simulink model "ModelForSlidesFeb"  (R2023a)
settings: Solver=VariableStepAuto  StartTime=0  StopTime=1000  FixedStep=0.01  RelTol=1e-3
model workspace (MAT data in the model file):
  finalint = 0
  firstWarning = 1
  originalScenarioChecksum = '114339432DE22364D47BB28FC96DC10C'
undefined symbols (not defined in the file): Acceleration, ActorID, AngularVelocity, curvature, DefaultGear, Defined, DEND_B, DEND_S, DEND_T, direction, DiscIntNeverNeededParam, driving, Ego, gradbp, L, Lane, LF, LR, m, matlabshared, MAX_BRAKE, MAX_STEER, MAX_TORQUE, maxNumActors, MCAR, MIN_BRAKE, MIN_STEER, MIN_TORQUE, n, NUMD_B, NUMD_S, NUMD_T, Pitch, Pose, Position, psi_o, R, Roll, RRdamp, SceneInfo, session, sigbuilder_block, STEER_RATIO, stopSign_ID, Tdead, thetaRefs, TL_ID, TrackWidth, ts, Ts, User, Vdead, Velocity, WB, X_o, xRef2s, Y_o, Yaw, yRef2s
libraries: drivingscenarioandsensors x13, roadrunnerscenario x11, simulink x8, simulink_extras x5, drivingvehiclecontroller x2, trackingutilitieslib x2, robotalgslib x1, mpcadaslib x1, slpidlib x1, drivinglib x1, autolibshared x1, vehdynlibviscommon x1
(part 1 of 4)
settings Model: Creator=akshran  LastModifiedBy=almudhaf.3
settings DataIOCC: SignalLogging=off
settings OptimizationCC: ReuseModelBlockBuffer=off
settings DebuggingCC: UnconnectedInputMsg=warning  UnconnectedOutputMsg=warning  UnconnectedLineMsg=warning  UnderSpecifiedDimensionMsg=warning
settings ModelReferenceCC: EnableRefExpFcnMdlSchedulingChecks=on
settings RTWCC: DLArmComputeVersion=19.05

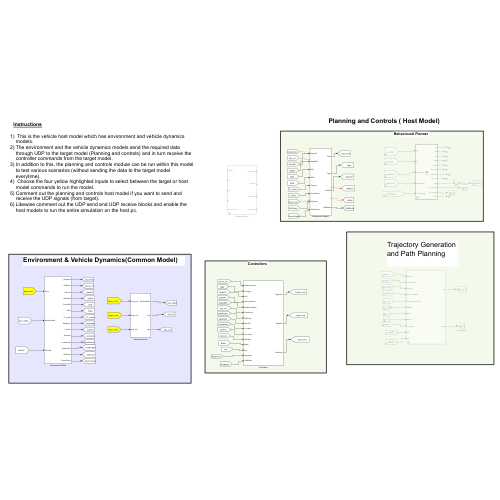
[thumbnail: Simulink's stored preview of the top-level diagram]
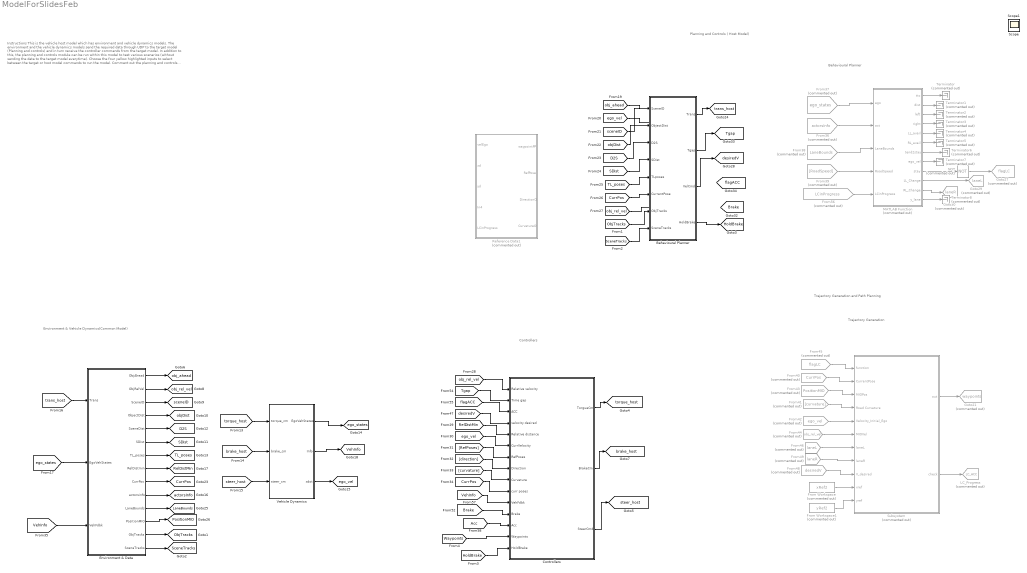
== system ModelForSlidesFeb ==
  note: Trajectory Generation and Path Planning
  note: Trajectory Generation
  note: Behavioural Planner
  note: Instructions
      |
      | This is the vehicle host model which has environment and vehicle dynamics models.
      | The environment and the vehicle dynamics models send the required data through UDP to the target model (Planning and controls) and in turn receive the controller commands from the target model.
      | In addition to this, the planning and controls module can be run within this model to test various scenarios (without sending the data to the target model everytime).
      | Choose the four yellow highlighted inputs to select between the target or host model commands to run the model.
      | Comment out the planning and controls host model if you want to send and receive the UDP signals (from target).
      | Likewise comment out the UDP send and UDP receive blocks and enable the host models to run the entire simulation on the host pc.
  note: Environment & Vehicle Dynamics(Common Model)
  note: Planning and Controls ( Host Model)
  note: Controllers
  Behavioural Planner : Subsystem
  Controllers : Subsystem
  Environment & Data : Subsystem
  From Workspace : FromWorkspace  Commented=on  VariableName=xRef2
  From Workspace1 : FromWorkspace  Commented=on  VariableName=yRef2
  From36 : From  Commented=on  GotoTag=actorsInfo  TagVisibility=global
  From37 : From  Commented=on  GotoTag=ego_states  TagVisibility=global
  From38 : From  Commented=on  GotoTag=LaneBounds  TagVisibility=global
  From39 : From  Commented=on  GotoTag=RoadSpeed  TagVisibility=global
  From40 : From  Commented=on  GotoTag=CurrPos  TagVisibility=global
  From41 : From  Commented=on  GotoTag=curvature
  From42 : From  Commented=on  GotoTag=ego_vel  TagVisibility=global
  From43 : From  Commented=on  GotoTag=PositionMIO  TagVisibility=global
  From44 : From  Commented=on  GotoTag=obj_rel_vel  TagVisibility=global
  From45 : From  Commented=on  GotoTag=flagLC  TagVisibility=global
  From46 : From  Commented=on  GotoTag=laneL  TagVisibility=global
  From48 : From  Commented=on  GotoTag=desiredV  TagVisibility=global
  From49 : From  Commented=on  GotoTag=laneR  TagVisibility=global
  From56 : From  Commented=on  GotoTag=LCinProgress  TagVisibility=global
  Goto21 : Goto  Commented=on  GotoTag=waypoints  TagVisibility=global
  Goto27 : Goto  Commented=on  GotoTag=flagLC  TagVisibility=global
  Goto29 : Goto  Commented=on  GotoTag=laneL  TagVisibility=global
  Goto30 : Goto  Commented=on  GotoTag=laneR  TagVisibility=global
  LC_Progress : Goto  Commented=on  GotoTag=LC_ACC  TagVisibility=global
  MATLAB Function : MATLAB Function  Commented=on  TreatAsAtomicUnit=on
  NOT : Logic  Commented=on  Operator=NOT  IconShape=distinctive  AllPortsSameDT=off  OutDataTypeStr=boolean
  Reference Data1 : Subsystem  Commented=on  VariantControl=Stanley
  Subsystem : Subsystem  Commented=on
  Terminator{,1..8} (9 alike) : Terminator  Commented=on
  Vehicle Dynamics : Subsystem
  Scope : Scope
  Scope1 : Scope
  tag scope: Brake=global, CurrPos=global, D2S=global, HoldBrake=global, LaneBounds=global, ObjTracks=global, PositionMIO=global, RelDistMin=global, SDist=global, SceneTracks=global, TL_poses=global, Tgap=global, VehInfo=global, actorsInfo=global, brake_host=global, desiredV=global, ego_states=global, ego_vel=global, flagACC=global, objDist=global, obj_ahead=global, obj_rel_vel=global, sceneID=global, steer_host=global, torque_host=global, trans_host=global
  wires:
  Controllers/1(TorgueCm) -> [torque_host]
  Environment & Data/1(ObjAhead) -> [obj_ahead]
  Environment & Data/2(ObjRelVel) -> [obj_rel_vel]
  Environment & Data/3(SceneID) -> [sceneID]
  Environment & Data/4(ObjectDist) -> [objDist]
  Environment & Data/6(SDist) -> [SDist]
  Environment & Data/5(SceneDist) -> [D2S]
  Environment & Data/7(TL_poses) -> [TL_poses]
  Vehicle Dynamics/1(EgoVehStates) -> [ego_states]
  Vehicle Dynamics/3(xdot) -> [ego_vel]
  Environment & Data/8(RelDistmin) -> [RelDistMin]
  Vehicle Dynamics/2(Info) -> [VehInfo]
  [torque_host] -> Vehicle Dynamics/1(torque_cm)
  [brake_host] -> Vehicle Dynamics/2(brake_cm)
  [steer_host] -> Vehicle Dynamics/3(steer_cm)
  [trans_host] -> Environment & Data/1(Trans)
  [ego_states] -> Environment & Data/2(EgoVehStates)
  [obj_rel_vel] -> Controllers/1(Relative velocity)
  [RelDistMin] -> Controllers/5(Relative distance)
  [ego_vel] -> Controllers/6(CurrVelocity)
  [RefPoses] -> Controllers/7(RefPoses)
  [direction] -> Controllers/8(Direction)
  [curvature] -> Controllers/9(Curvature)
  [CurrPos] -> Controllers/10(curr poses)
  [VehInfo] -> Environment & Data/3(VehFdbk)
  Environment & Data/9(CurrPos) -> [CurrPos]
  Environment & Data/10(actorsinfo) -> [actorsInfo]
  From37/1 -> MATLAB Function/1(ego)
  From36/1 -> MATLAB Function/2(act)
  Environment & Data/11(LaneBounds) -> [LaneBounds]
  From38/1 -> MATLAB Function/3(LaneBounds)
  From39/1 -> MATLAB Function/4(RoadSpeed)
  MATLAB Function/9(stay) -> NOT/1
  MATLAB Function/10(LL_Change) -> Goto29/1
  MATLAB Function/11(RL_Change) -> Goto30/1
  Environment & Data/12(PositionMIO) -> [PositionMIO]
  NOT/1 -> Goto27/1
  [desiredV] -> Controllers/4(velocity desired)
  [Tgap] -> Controllers/2(Time gap)
  [flagACC] -> Controllers/3(ACC)
  From56/1 -> MATLAB Function/5(LCinProgress)
  [VehInfo] -> Controllers/11(VehFdbk)
  Controllers/2(BrakeCm) -> [brake_host]
  Controllers/3(SteerCmd) -> [steer_host]
  From45/1 -> Subsystem/1(function)
  From40/1 -> Subsystem/2(CurrentPose)
  From43/1 -> Subsystem/3(MIOPos)
  From41/1 -> Subsystem/4(Road Curvature)
  From42/1 -> Subsystem/5(Velocity_Initial_Ego)
  From44/1 -> Subsystem/6(MIOVel)
  From48/1 -> Subsystem/9(V_desired)
  Subsystem/2(check) -> LC_Progress/1
  [obj_ahead] -> ?
  [ego_vel] -> ?
  [sceneID] -> Behavioural Planner/1(SceneID)
  [objDist] -> Behavioural Planner/2(ObjectDist)
  [D2S] -> Behavioural Planner/3(D2S)
  [SDist] -> Behavioural Planner/4(SDist)
  [TL_poses] -> Behavioural Planner/5(TLposes)
  [CurrPos] -> Behavioural Planner/6(CurrentPose)
  [obj_rel_vel] -> ?
  Behavioural Planner/1(Trans) -> [trans_host]
  Behavioural Planner/2(Tgap) -> [Tgap]
  Behavioural Planner/3(VelCmd) -> [desiredV]
  ? -> [flagACC]
  ? -> [Brake]
  [Brake] -> Controllers/12(Brake)
  [Acc] -> Controllers/13(Acc)
  Subsystem/1(out) -> Goto21/1
  From46/1 -> Subsystem/7(laneL)
  From49/1 -> Subsystem/8(laneR)
  From Workspace/1 -> Subsystem/10(xref)
  From Workspace1/1 -> Subsystem/11(yref)
  MATLAB Function/1(ttc) -> Terminator/1
  MATLAB Function/2(dist) -> Terminator1/1
  MATLAB Function/3(left) -> Terminator2/1
  MATLAB Function/4(right) -> Terminator3/1
  MATLAB Function/5(LL_avail) -> Terminator4/1
  MATLAB Function/6(RL_avail) -> Terminator5/1
  MATLAB Function/7(tend2stay) -> Terminator6/1
  MATLAB Function/8(ego_vel) -> Terminator7/1
  MATLAB Function/12(y_lane) -> Terminator8/1
  Environment & Data/14(SceneTracks) -> [SceneTracks]
  Environment & Data/13(ObjTracks) -> [ObjTracks]
  [ObjTracks] -> Behavioural Planner/7(ObjTracks)
  [SceneTracks] -> Behavioural Planner/8(SceneTracks)
  Behavioural Planner/4(HoldBrake) -> [HoldBrake]
  [HoldBrake] -> Controllers/15(HoldBrake)
  [Waypoints] -> Controllers/14(Waypoints)

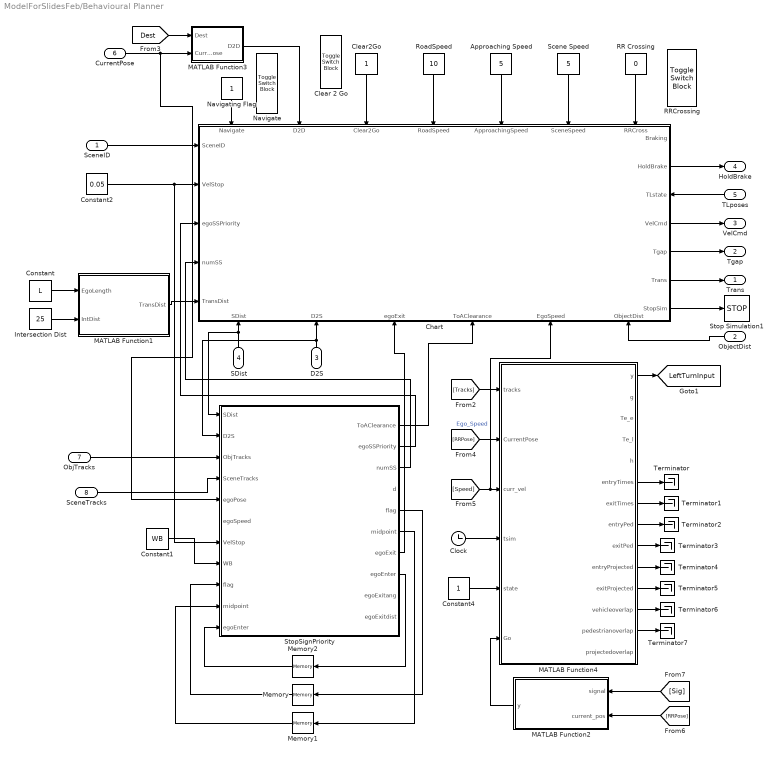
== system ModelForSlidesFeb/Behavioural Planner ==
  SceneID : Inport
  ObjectDist : Inport  Port=2
  D2S : Inport  Port=3
  SDist : Inport  Port=4
  TLposes : Inport  Port=5
  CurrentPose : Inport  Port=6
  ObjTracks : Inport  Port=7
  SceneTracks : Inport  Port=8
  Approaching Speed : Constant  Value=5
  Chart : Stateflow chart  TreatAsAtomicUnit=on
      settings: PortSchema="{\"entries\":[{\"content\":{\"sides\":[{\"content\":{\"connectorIds\":[\"In17\",\"In18\",\"In19\",\"In2\",\"In5\"]},\"type\":\"ConnectorPlacement.EquallySpacedRectSide\",\"uuid\":\"81aca70f-0947-49fb-b60a-be241e44193b\"},{\"content\":{\"connectorIds\":[\"Out6\",\"Out2\",\"In1\",\"Out1\",\"Out3\",\"Out4\",\"Out5\"],\"side\":\"RIGHT\"},\"type\":\"ConnectorPlacement.EquallySpacedRectSide\",\"uuid\":\"e7b9645e-3711-4964-ac9b-0199dd335e99\"},{\"content\":{\"connectorIds\":[\"In13\",\"In14\",\"In15\",\"In16\",\"In6\",\"In9\",\"In11\"],\"side\":\"TOP\"},\"type\":\"ConnectorPlacement.EquallySpacedRectSide\",\"uuid\":\"6876f024-944b-4540-9404-d68f37763657\"},{\"content\":{\"connectorIds\":[\"In10\",\"In12\",\"In3\",\"In4\",\"In7\",\"In8\"],\"side\":\"BOTTOM\"},\"type\":\"ConnectorPlacement.EquallySpacedRectSide\",\"uuid\":\"44acab73-cdde-4edf-95df-27422644ccab\"}]},\"type\":\"ConnectorPlacement.EquallySpacedConnector\",\"uuid\":\"d2c31c01-e447-43db-8d2b-8b98a0ca291a\"}],\"packageUris\":[\"http://schema.mathworks.com/mf0/Connector/R2020b\"],\"version\":\"1.0\"}"
  Clear 2 Go : ToggleSwitchBlock
      settings: Values={{'Off', 'On'}, [0 1]}
  Clear2Go : Constant
  Clock : Clock
  Constant : Constant  Value=L
  Constant1 : Constant  Value=WB
  Constant2 : Constant  Value=0.05
  Constant4 : Constant
  Intersection Dist : Constant  Value=25
  MATLAB Function1 : MATLAB Function  TreatAsAtomicUnit=on
  MATLAB Function2 : MATLAB Function  TreatAsAtomicUnit=on
  MATLAB Function3 : MATLAB Function  TreatAsAtomicUnit=on
  MATLAB Function4 : MATLAB Function  TreatAsAtomicUnit=on
  Memory : Memory
  Memory1 : Memory  InitialCondition=[0 0]
  Memory2 : Memory
  Navigate : ToggleSwitchBlock
      settings: Values={{'Off', 'On'}, [0 1]}
  Navigating Flag : Constant
  RR Crossing : Constant  Value=0
  RRCrossing : ToggleSwitchBlock
      settings: Values={{'Off', 'On'}, [0 1]}
  RoadSpeed : Constant  Value=10
  Scene Speed : Constant  Value=5
  Stop Simulation1 : Stop
  StopSignPriority : MATLAB Function  TreatAsAtomicUnit=on
  Terminator{,1..7} (8 alike) : Terminator
  Trans : Outport
  Tgap : Outport  Port=2
  VelCmd : Outport  Port=3
  HoldBrake : Outport  Port=4
  tag scope: LeftTurnInput=global
  wires:
  Clear2Go/1 -> Chart/15(Clear2Go)
  ObjectDist/1 -> Chart/8(ObjectDist)
  Navigating Flag/1 -> Chart/13(Navigate)
  Approaching Speed/1 -> Chart/6(ApproachingSpeed)
  Scene Speed/1 -> Chart/9(SceneSpeed)
  CurrentPose/1 -> StopSignPriority/5(egoPose), MATLAB Function3/2(CurrentPose)
  RR Crossing/1 -> Chart/11(RRCross)
  RoadSpeed/1 -> Chart/16(RoadSpeed)
  SceneID/1 -> Chart/17(SceneID)
  Chart/5(StopSim) -> Stop Simulation1/1
  Chart/4(Trans) -> Trans/1
  TLposes/1 -> Chart/1(TLstate)
  Chart/1(VelCmd) -> VelCmd/1
  SDist/1 -> StopSignPriority/1(SDist), Chart/10(SDist)
  D2S/1 -> Chart/12(D2S), StopSignPriority/2(D2S)
  Chart/3(Tgap) -> Tgap/1
  Constant/1 -> MATLAB Function1/1(EgoLength)
  Intersection Dist/1 -> MATLAB Function1/2(IntDist)
  MATLAB Function1/1(TransDist) -> Chart/5(TransDist)
  MATLAB Function3/1(D2D) -> Chart/14(D2D)
  Constant2/1 -> StopSignPriority/7(VelStop), Chart/18(VelStop)
  StopSignPriority/2(egoSSPriority) -> Chart/19(egoSSPriority)
  SceneTracks/1 -> StopSignPriority/4(SceneTracks)
  ObjTracks/1 -> StopSignPriority/3(ObjTracks)
  StopSignPriority/3(numSS) -> Chart/2(numSS)
  Constant1/1 -> StopSignPriority/8(WB)
  Memory/1 -> StopSignPriority/9("flag ")
  StopSignPriority/5(flag) -> Memory/1
  StopSignPriority/6(midpoint) -> Memory1/1
  Memory1/1 -> StopSignPriority/10("midpoint ")
  StopSignPriority/7(egoExit) -> Chart/3(egoExit)
  StopSignPriority/1(ToAClearance) -> Chart/4(ToAClearance)
  Chart/2(HoldBrake) -> HoldBrake/1
  StopSignPriority/8(egoEnter) -> Memory2/1
  Memory2/1 -> StopSignPriority/11("egoEnter ")
  [Dest] -> MATLAB Function3/1(Dest)
  [RRPose] -> MATLAB Function2/2(current_pos)
  MATLAB Function4/6(entryTimes) -> Terminator/1
  [Speed] -> Chart/7(EgoSpeed), MATLAB Function4/3(curr_vel)  "Ego_Speed"
  MATLAB Function4/13(pedestrianoverlap) -> Terminator7/1
  MATLAB Function4/1(y) -> [LeftTurnInput]
  MATLAB Function4/8(entryPed) -> Terminator2/1
  MATLAB Function4/11(exitProjected) -> Terminator5/1
  MATLAB Function4/9(exitPed) -> Terminator3/1
  Clock/1 -> MATLAB Function4/4(tsim)
  MATLAB Function4/12(vehicleoverlap) -> Terminator6/1
  MATLAB Function4/7(exitTimes) -> Terminator1/1
  MATLAB Function2/1(y) -> MATLAB Function4/6(Go)
  [Tracks] -> MATLAB Function4/1(tracks)
  [Sig] -> MATLAB Function2/1(signal)
  MATLAB Function4/10(entryProjected) -> Terminator4/1
  [RRPose] -> MATLAB Function4/2(CurrentPose)
  Constant4/1 -> MATLAB Function4/5(state)

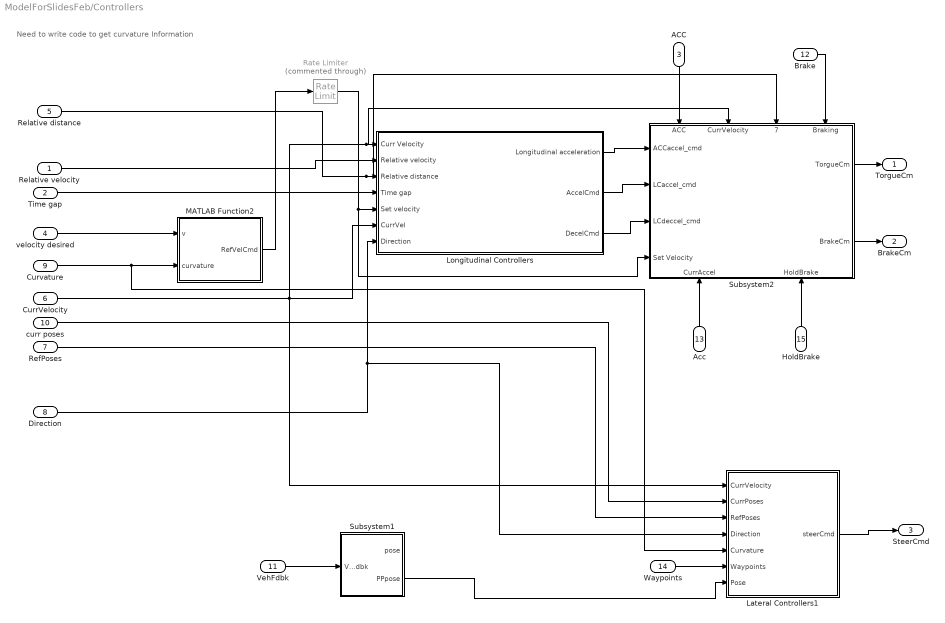
== system ModelForSlidesFeb/Controllers ==
  note: Need to write code to get curvature Information
  Relative velocity : Inport
  Time gap : Inport  Port=2
  ACC : Inport  Port=3
  velocity desired : Inport  Port=4
  Relative distance : Inport  Port=5
  CurrVelocity : Inport  Port=6
  RefPoses : Inport  Port=7
  Direction : Inport  Port=8
  Curvature : Inport  Port=9
  curr poses : Inport  Port=10
  VehFdbk : Inport  Port=11
  Brake : Inport  Port=12
  Acc : Inport  Port=13
  Waypoints : Inport  Port=14
  HoldBrake : Inport  Port=15
  Lateral Controllers1 : Subsystem
  Longitudinal Controllers : Subsystem
  MATLAB Function2 : MATLAB Function  TreatAsAtomicUnit=on
  Rate Limiter : RateLimiter  Commented=through  RisingSlewLimit=2  SampleTimeMode=inherited
  Subsystem1 : Subsystem
  Subsystem2 : Subsystem
      settings: PortSchema="{\"entries\":[{\"content\":{\"sides\":[{\"content\":{\"connectorIds\":[\"In1\",\"In2\",\"In3\",\"In4\"]},\"type\":\"ConnectorPlacement.EquallySpacedRectSide\",\"uuid\":\"a23b1a10-3bcb-40a0-900c-c9a3f160b173\"},{\"content\":{\"connectorIds\":[\"Out1\",\"Out2\"],\"side\":\"RIGHT\"},\"type\":\"ConnectorPlacement.EquallySpacedRectSide\",\"uuid\":\"88840b66-912f-4184-aeec-297642319416\"},{\"content\":{\"connectorIds\":[\"In5\",\"In6\",\"In7\",\"In8\"],\"side\":\"TOP\"},\"type\":\"ConnectorPlacement.EquallySpacedRectSide\",\"uuid\":\"37a03ca9-b065-473e-b290-3b07703c6005\"},{\"content\":{\"connectorIds\":[\"In9\",\"In10\"],\"side\":\"BOTTOM\"},\"type\":\"ConnectorPlacement.EquallySpacedRectSide\",\"uuid\":\"275ca825-7815-497a-af18-67b3ec4705b4\"}]},\"type\":\"ConnectorPlacement.EquallySpacedConnector\",\"uuid\":\"5bfc7c71-8f7a-4cba-a168-7eeca22a2fcb\"}],\"packageUris\":[\"http://schema.mathworks.com/mf0/Connector/R2020b\"],\"version\":\"1.0\"}"
  TorgueCm : Outport
  BrakeCm : Outport  Port=2
  SteerCmd : Outport  Port=3
  wires:
  Curvature/1 -> MATLAB Function2/2(curvature), Lateral Controllers1/5(Curvature)
  Relative velocity/1 -> Longitudinal Controllers/2(Relative velocity)
  MATLAB Function2/1(RefVelCmd) -> Rate Limiter/1
  Direction/1 -> Longitudinal Controllers/7(Direction), Lateral Controllers1/4(Direction)
  RefPoses/1 -> Lateral Controllers1/3(RefPoses)
  velocity desired/1 -> MATLAB Function2/1(v)
  CurrVelocity/1 -> Subsystem2/6(CurrVelocity), Longitudinal Controllers/1(Curr Velocity), Longitudinal Controllers/6(CurrVel), Lateral Controllers1/1(CurrVelocity)
  Time gap/1 -> Longitudinal Controllers/4(Time gap)
  Relative distance/1 -> Subsystem2/7(Relative Distance), Longitudinal Controllers/3(Relative distance)
  Subsystem1/2(PPpose) -> Lateral Controllers1/7(Pose)
  VehFdbk/1 -> Subsystem1/1(VehFdbk)
  Lateral Controllers1/1(steerCmd) -> SteerCmd/1
  Rate Limiter/1 -> Subsystem2/4(Set Velocity), Longitudinal Controllers/5(Set velocity)
  curr poses/1 -> Lateral Controllers1/2(CurrPoses)
  Longitudinal Controllers/1(Longitudinal acceleration) -> Subsystem2/1(ACCaccel_cmd)
  Longitudinal Controllers/2(AccelCmd) -> Subsystem2/2(LCaccel_cmd)
  Longitudinal Controllers/3(DecelCmd) -> Subsystem2/3(LCdeccel_cmd)
  ACC/1 -> Subsystem2/5(ACC)
  Subsystem2/1(TorgueCm) -> TorgueCm/1
  Subsystem2/2(BrakeCm) -> BrakeCm/1
  Acc/1 -> Subsystem2/9(CurrAccel)
  Brake/1 -> Subsystem2/8(Braking)
  Waypoints/1 -> Lateral Controllers1/6(Waypoints)
  HoldBrake/1 -> Subsystem2/10(HoldBrake)

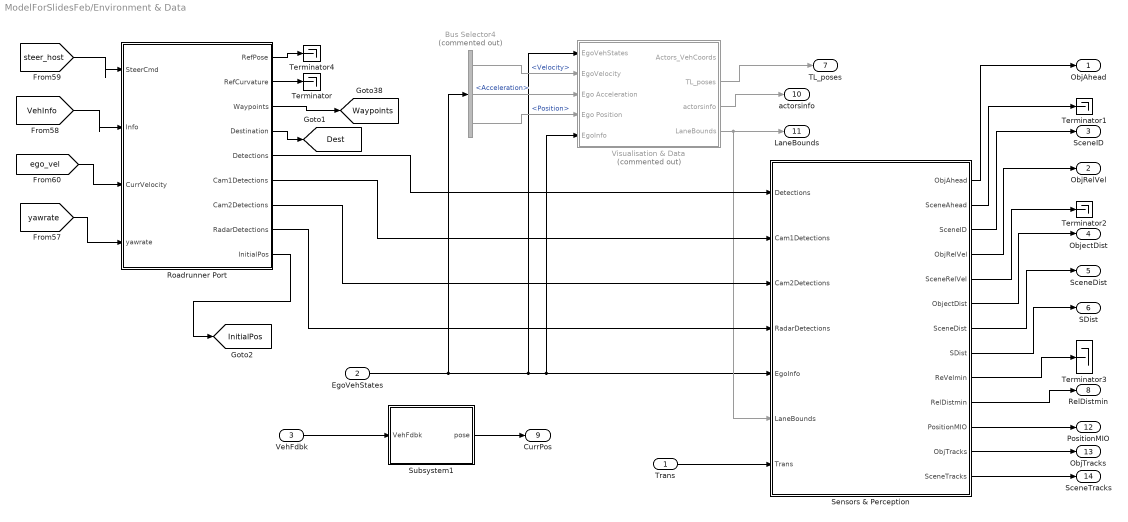
== system ModelForSlidesFeb/Environment & Data ==
  Trans : Inport
  EgoVehStates : Inport  Port=2
  VehFdbk : Inport  Port=3
  Bus Selector4 : BusSelector  Commented=on  OutputSignals=Velocity,Acceleration,Position
  Roadrunner Port : Subsystem
  Sensors & Perception : Subsystem
  Subsystem1 : Subsystem
  Terminator{,1..4} (5 alike) : Terminator
  Visualisation & Data : Subsystem  Commented=on
  ObjAhead : Outport
  ObjRelVel : Outport  Port=2
  SceneID : Outport  Port=3
  ObjectDist : Outport  Port=4
  SceneDist : Outport  Port=5
  SDist : Outport  Port=6
  TL_poses : Outport  Port=7
  RelDistmin : Outport  Port=8
  CurrPos : Outport  Port=9
  actorsinfo : Outport  Port=10
  LaneBounds : Outport  Port=11
  PositionMIO : Outport  Port=12
  ObjTracks : Outport  Port=13
  SceneTracks : Outport  Port=14
  tag scope: Dest=global, InitialPos=global, Waypoints=global
  wires:
  Sensors & Perception/11(PositionMIO) -> PositionMIO/1
  Sensors & Perception/3(SceneID) -> SceneID/1
  Subsystem1/1(pose) -> CurrPos/1
  Sensors & Perception/5(SceneRelVel) -> Terminator2/1
  EgoVehStates/1 -> Bus Selector4/1, Visualisation & Data/1(EgoVehStates), Visualisation & Data/5(EgoInfo), Sensors & Perception/5(EgoInfo)
  VehFdbk/1 -> Subsystem1/1(VehFdbk)
  Bus Selector4/2 -> Visualisation & Data/3(Ego Acceleration)  "<Acceleration>"
  Bus Selector4/1 -> Visualisation & Data/2(EgoVelocity)  "<Velocity>"
  Visualisation & Data/2(TL_poses) -> TL_poses/1
  Bus Selector4/3 -> Visualisation & Data/4(Ego Position)  "<Position>"
  Visualisation & Data/3(actorsinfo) -> actorsinfo/1
  Visualisation & Data/4(LaneBounds) -> LaneBounds/1, Sensors & Perception/6(LaneBounds)
  Trans/1 -> Sensors & Perception/7(Trans)
  Sensors & Perception/9(ReVelmin) -> Terminator3/1
  Sensors & Perception/1(ObjAhead) -> ObjAhead/1
  Sensors & Perception/10(RelDistmin) -> RelDistmin/1
  Sensors & Perception/2(SceneAhead) -> Terminator1/1
  Sensors & Perception/4(ObjRelVel) -> ObjRelVel/1
  Sensors & Perception/6(ObjectDist) -> ObjectDist/1
  Sensors & Perception/7(SceneDist) -> SceneDist/1
  Sensors & Perception/8(SDist) -> SDist/1
  Sensors & Perception/12(ObjTracks) -> ObjTracks/1
  Sensors & Perception/13(SceneTracks) -> SceneTracks/1
  [ego_vel] -> Roadrunner Port/3(CurrVelocity)
  [yawrate] -> Roadrunner Port/4(yawrate)
  Roadrunner Port/3(Waypoints) -> [Waypoints]
  Roadrunner Port/4(Destination) -> [Dest]
  [VehInfo] -> Roadrunner Port/2(Info)
  [steer_host] -> Roadrunner Port/1(SteerCmd)
  Roadrunner Port/5(Detections) -> Sensors & Perception/1(Detections)
  Roadrunner Port/2(RefCurvature) -> Terminator/1
  Roadrunner Port/1(RefPose) -> Terminator4/1
  Roadrunner Port/6(Cam1Detections) -> Sensors & Perception/2(Cam1Detections)
  Roadrunner Port/7(Cam2Detections) -> Sensors & Perception/3(Cam2Detections)
  Roadrunner Port/8(RadarDetections) -> Sensors & Perception/4(RadarDetections)
  Roadrunner Port/9(InitialPos) -> [InitialPos]

== system ModelForSlidesFeb/Reference Data1 ==
  velEgo : Inport
  xd : Inport  Port=2
  yd : Inport  Port=3
  In4 : Inport  Port=4
  LCinProgress : Inport  Port=5
  Discrete-Time Integrator : DiscreteIntegrator  SampleTime=-1  ICPrevOutput=DiscIntNeverNeededParam  ICPrevScaledInput=DiscIntNeverNeededParam
  Memory : Memory
  Memory1 : Memory
  Merge : Merge
  Merge1 : Merge
  Subsystem : Subsystem
  Subsystem1 : Subsystem
  Subsystem2 : Subsystem
  Subsystem3 : Subsystem
  Switch : Switch  Criteria=u2 ~= 0  SaturateOnIntegerOverflow=off  InputSameDT=off
  Switch Case : SwitchCase  CaseConditions={1,0}  ShowDefaultCase=off
  waypointPP : Outport
  RefPose : Outport  Port=2
  DirectionO : Outport  Port=3
  CurvatureO : Outport  Port=4
  wires:
  velEgo/1 -> Subsystem3/1(VelFdbk), Subsystem2/1(VelFdbk), Discrete-Time Integrator/1
  Subsystem2/4(WayPoints) -> Merge1/1
  Merge1/1 -> waypointPP/1
  Subsystem2/1(RefPose) -> Switch/3
  Subsystem2/2(DirectionO) -> DirectionO/1
  Merge/1 -> CurvatureO/1
  Subsystem2/3(CurvatureO) -> Merge/2
  Subsystem3/1(RefPose) -> Switch/1
  Switch Case/1 -> Subsystem3/Action
  Switch Case/2 -> Subsystem2/Action
  xd/1 -> Memory/1
  yd/1 -> Memory1/1
  Memory/1 -> Subsystem3/2(xd)
  Memory1/1 -> Subsystem3/4(yd)
  Subsystem2/5(finalint) -> Subsystem3/3(finalint)
  Subsystem/1(Out1) -> Switch/2, Switch Case/1, Subsystem1/2(enable)
  LCinProgress/1 -> Subsystem/Enable
  Discrete-Time Integrator/1 -> Subsystem1/1(Integrator)
  Subsystem1/1(Ref pose) -> RefPose/1

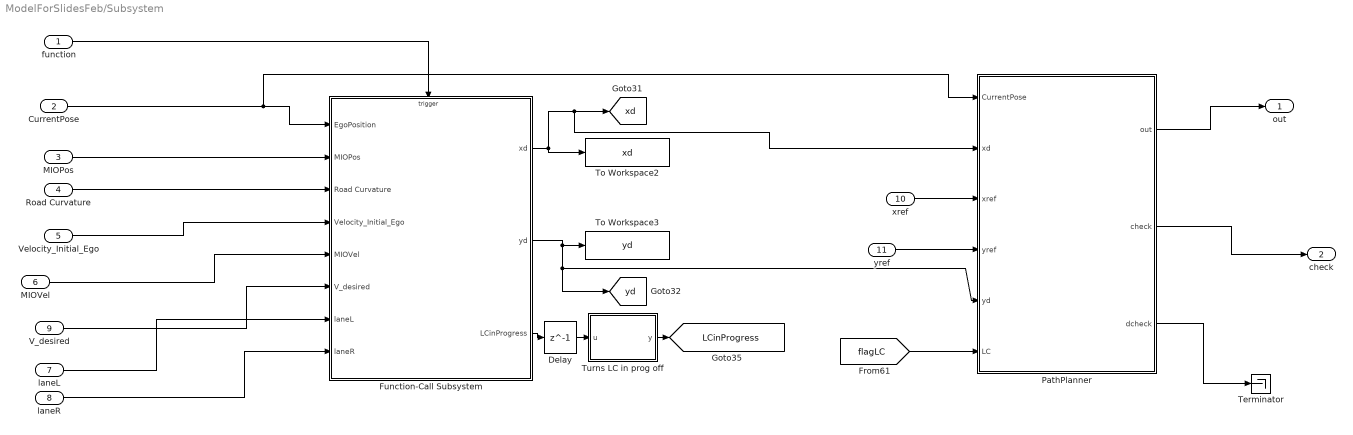
== system ModelForSlidesFeb/Subsystem ==
  function : Inport
  CurrentPose : Inport  Port=2
  MIOPos : Inport  Port=3
  Road Curvature : Inport  Port=4
  Velocity_Initial_Ego : Inport  Port=5
  MIOVel : Inport  Port=6
  laneL : Inport  Port=7
  laneR : Inport  Port=8
  V_desired : Inport  Port=9
  xref : Inport  Port=10
  yref : Inport  Port=11
  Delay : Delay  DelayLength=1
  Function-Call Subsystem : Subsystem  TreatAsAtomicUnit=on
  PathPlanner : Subsystem
  Terminator : Terminator
  To Workspace2 : ToWorkspace  VariableName=xd  SampleTime=-1
      settings: Save2DSignal=2-D array (concatenate along first dimension)
  To Workspace3 : ToWorkspace  VariableName=yd  SampleTime=-1
      settings: Save2DSignal=2-D array (concatenate along first dimension)
  Turns LC in prog off : MATLAB Function  TreatAsAtomicUnit=on
  out : Outport
  check : Outport  Port=2
  tag scope: LCinProgress=global, xd=global, yd=global
  wires:
  MIOVel/1 -> Function-Call Subsystem/5(MIOVel)
  Road Curvature/1 -> Function-Call Subsystem/3(Road Curvature)
  PathPlanner/1(out) -> out/1
  PathPlanner/2(check) -> check/1
  Velocity_Initial_Ego/1 -> Function-Call Subsystem/4(Velocity_Initial_Ego)
  V_desired/1 -> Function-Call Subsystem/6(V_desired)
  MIOPos/1 -> Function-Call Subsystem/2(MIOPos)
  Function-Call Subsystem/1(xd) -> To Workspace2/1, PathPlanner/2(xd), [xd]
  Function-Call Subsystem/2(yd) -> PathPlanner/5(yd), [yd], To Workspace3/1
  Delay/1 -> Turns LC in prog off/1(u)
  Turns LC in prog off/1(y) -> [LCinProgress]
  Function-Call Subsystem/3(LCinProgress) -> Delay/1
  CurrentPose/1 -> PathPlanner/1(CurrentPose), Function-Call Subsystem/1(EgoPosition)
  function/1 -> Function-Call Subsystem/Trigger
  laneL/1 -> Function-Call Subsystem/7(laneL)
  laneR/1 -> Function-Call Subsystem/8(laneR)
  xref/1 -> PathPlanner/3(xref)
  yref/1 -> PathPlanner/4(yref)
  PathPlanner/3(dcheck) -> Terminator/1
  [flagLC] -> PathPlanner/6(LC)

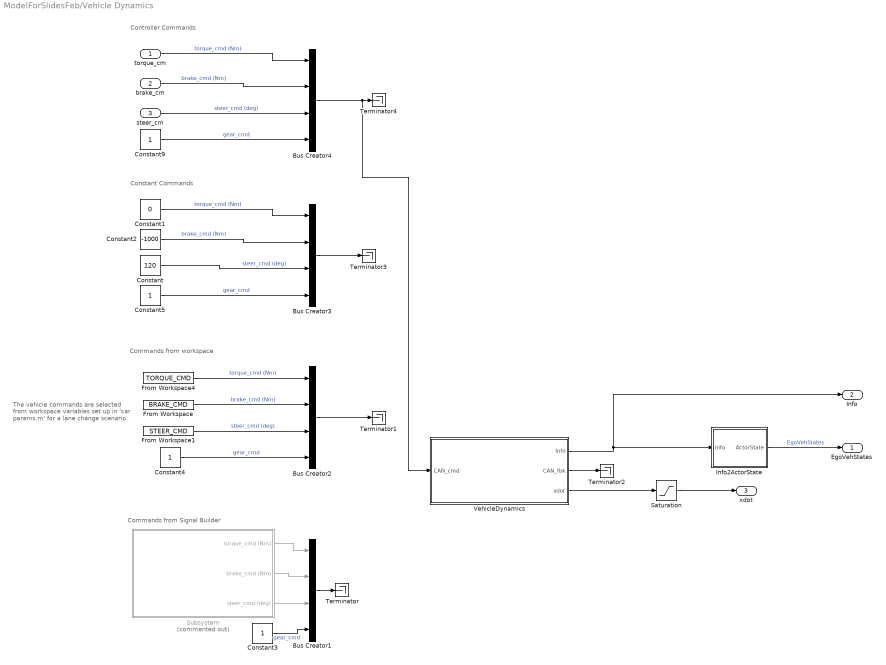
== system ModelForSlidesFeb/Vehicle Dynamics ==
  note: Constant Commands
  note: Commands from workspace
  note: Commands from Signal Builder
  note: The vehicle commands are selected from workspace variables set up in 'car params.m' for a lane change scenario
  note: Controller Commands
  torque_cm : Inport
  brake_cm : Inport  Port=2
  steer_cm : Inport  Port=3
  Bus Creator{1..4} (4 alike) : BusCreator  Inputs=4
  Constant : Constant  Value=120
  Constant1 : Constant  Value=0
  Constant2 : Constant  Value=-1000
  Constant{3..5,9} (4 alike) : Constant
  From Workspace : FromWorkspace  VariableName=BRAKE_CMD  SampleTime=ts
  From Workspace1 : FromWorkspace  VariableName=STEER_CMD  SampleTime=ts
  From Workspace4 : FromWorkspace  VariableName=TORQUE_CMD  SampleTime=ts
  Info2ActorState : Subsystem
  Saturation : Saturate  UpperLimit=inf  LowerLimit=0.001
  Subsystem : Subsystem  Commented=on
  Terminator{,1..4} (5 alike) : Terminator
  VehicleDynamics : Subsystem  mask{InitPosition=[X_o Y_o 0]*0, InitSpeed=0, InitYaw=psi_o}
      mask prompts: InitPosition "Initial Position (m)"; InitSpeed "Initial Speed (m/s)"; InitYaw "Init Yaw (rad)"
  EgoVehStates : Outport
  Info : Outport  Port=2
  xdot : Outport  Port=3
  wires:
  Bus Creator2/1 -> Terminator1/1
  VehicleDynamics/2(CAN_fbk) -> Terminator2/1
  VehicleDynamics/1(Info) -> Info/1, Info2ActorState/1(Info)
  Constant/1 -> Bus Creator3/3  "steer_cmd (deg)"
  Info2ActorState/1(ActorState) -> EgoVehStates/1  "EgoVehStates"
  Constant1/1 -> Bus Creator3/1  "torque_cmd (Nm)"
  Constant2/1 -> Bus Creator3/2  "brake_cmd (Nm)"
  VehicleDynamics/3(xdot) -> Saturation/1
  Subsystem/1(torque_cmd (Nm)) -> Bus Creator1/1
  Subsystem/2(brake_cmd (Nm)) -> Bus Creator1/2
  Subsystem/3(steer_cmd (deg)) -> Bus Creator1/3
  Constant3/1 -> Bus Creator1/4  "gear_cmd"
  Constant4/1 -> Bus Creator2/4  "gear_cmd"
  From Workspace/1 -> Bus Creator2/2  "brake_cmd (Nm)"
  From Workspace1/1 -> Bus Creator2/3  "steer_cmd (deg)"
  From Workspace4/1 -> Bus Creator2/1  "torque_cmd (Nm)"
  Constant5/1 -> Bus Creator3/4  "gear_cmd"
  Bus Creator1/1 -> Terminator/1
  brake_cm/1 -> Bus Creator4/2  "brake_cmd (Nm)"
  Constant9/1 -> Bus Creator4/4  "gear_cmd"
  torque_cm/1 -> Bus Creator4/1  "torque_cmd (Nm)"
  steer_cm/1 -> Bus Creator4/3  "steer_cmd (deg)"
  Bus Creator3/1 -> Terminator3/1
  Bus Creator4/1 -> VehicleDynamics/1(CAN_cmd), Terminator4/1
  Saturation/1 -> xdot/1

== system ModelForSlidesFeb/Controllers/Lateral Controllers1 ==
  note: include toggle logic
  CurrVelocity : Inport
  CurrPoses : Inport  Port=2
  RefPoses : Inport  Port=3
  Direction : Inport  Port=4
  Curvature : Inport  Port=5
  Waypoints : Inport  Port=6
  Pose : Inport  Port=7
  Constant : Constant  Commented=on
  Demux : Demux  Commented=on  Outputs=3
  Demux1 : Demux  Commented=on  Outputs=3
  From : From  Commented=on  GotoTag=yawrate  TagVisibility=global
  Gain : Gain  Gain=1/STEER_RATIO
  Gain1 : Gain  Commented=on  Gain=180/pi
  Gain2 : Gain  Gain=180/pi
  Lateral Controller Stanley : drivingvehiclecontroller/Lateral Controller Stanley  Commented=on  ModelType=Kinematic bicycle model  PositionGainF=0.75  PositionGainR=2.5  YawRateGain=0.05  DelayGain=0.05  VehicleMass=MCAR  Lf=LF  Lr=LR  TireStiffness=5e3  Wheelbase=3  MaxSteeringAngle=30
  Pure Pursuit Controller1 : Subsystem
  Scope2 : Scope  Commented=on  NumInputPorts=2
  Unit Delay : UnitDelay  Commented=on  SampleTime=-1  HasFrameUpgradeWarning=on
  steerCmd : Outport
  wires:
  From/1 -> Gain1/1
  CurrPoses/1 -> Demux1/1, Lateral Controller Stanley/2
  Pure Pursuit Controller1/1(delta) -> Gain2/1
  Gain/1 -> steerCmd/1
  Curvature/1 -> ?
  CurrVelocity/1 -> Lateral Controller Stanley/3
  RefPoses/1 -> Demux/1, Lateral Controller Stanley/1
  Pose/1 -> Pure Pursuit Controller1/1(Pose)
  Lateral Controller Stanley/1 -> Unit Delay/1
  Constant/1 -> Lateral Controller Stanley/4
  Demux1/2 -> Scope2/2
  Demux/2 -> Scope2/1
  Gain2/1 -> Gain/1
  Waypoints/1 -> Pure Pursuit Controller1/2(Waypoints)

== system ModelForSlidesFeb/Controllers/Longitudinal Controllers ==
  Curr Velocity : Inport
  Relative velocity : Inport  Port=2
  Relative distance : Inport  Port=3
  Time gap : Inport  Port=4
  Set velocity : Inport  Port=5
  CurrVel : Inport  Port=6
  Direction : Inport  Port=7
  Adaptive Cruise Control System : mpcadaslib/Adaptive Cruise Control System  EgoModel=tf(1,[0.5,1,0])  InitialEgoVelocity=0  DefaultSpacing=WB+2  MaxVelocity=50  MinAcceleration=-40  amin_ext=off  MaxAcceleration=40  amax_ext=off  Ts=0.1  PredictionHorizon=10  ControllerBehavior=1.0  suboptimal=off  maxiter=10  datatypeopt=double  optmode=off  trackmode=off
  Constant : Constant
  Constant3 : Constant  Value=0
  Longitudinal Controller Stanley : drivingvehiclecontroller/Longitudinal Controller Stanley  Kp=5  Ki=2  SampleTime=0.05  MaxAcceleration=3.5  MaxDeceleration=2.4
  Longitudinal acceleration : Outport
  AccelCmd : Outport  Port=2
  DecelCmd : Outport  Port=3
  wires:
  Set velocity/1 -> Longitudinal Controller Stanley/1, Adaptive Cruise Control System/1
  Constant3/1 -> Longitudinal Controller Stanley/4
  Curr Velocity/1 -> Adaptive Cruise Control System/3
  CurrVel/1 -> Longitudinal Controller Stanley/2
  Longitudinal Controller Stanley/1 -> AccelCmd/1
  Longitudinal Controller Stanley/2 -> DecelCmd/1
  Relative velocity/1 -> Adaptive Cruise Control System/5
  Relative distance/1 -> Adaptive Cruise Control System/4
  Adaptive Cruise Control System/1 -> Longitudinal acceleration/1
  Time gap/1 -> Adaptive Cruise Control System/2
  Constant/1 -> Longitudinal Controller Stanley/3

== system ModelForSlidesFeb/Controllers/Subsystem1 ==
  VehFdbk : Inport
  Bus Selector : BusSelector  OutputSignals=InertFrm.Cg.Disp.X,InertFrm.Cg.Disp.Y,InertFrm.Cg.Ang.psi
  Bus Selector1 : BusSelector  Commented=on  OutputSignals=InertFrm.Cg.Disp.X,InertFrm.Cg.Disp.Y,InertFrm.Cg.Disp.Z
  Gain1 : Gain  Gain=180/pi
  Mux : Mux  Inputs=3
  Mux1 : Mux  Commented=on  Inputs=3
  Mux2 : Mux  Inputs=3
  Transpose : Math  Operator=transpose  SignedPower=on
  Transpose1 : Math  Commented=on  Operator=transpose  SignedPower=on
  Transpose2 : Math  Operator=transpose  SignedPower=on
  pose : Outport
  PPpose : Outport  Port=2
  wires:
  Mux/1 -> Transpose/1
  VehFdbk/1 -> Bus Selector1/1, Bus Selector/1
  Gain1/1 -> Mux/3
  Transpose/1 -> pose/1
  Bus Selector/3 -> Mux2/3, Gain1/1  "<psi>"
  Bus Selector1/1 -> Mux1/1  "<X>"
  Bus Selector1/2 -> Mux1/2  "<Y>"
  Bus Selector1/3 -> Mux1/3  "<Z>"
  Mux1/1 -> Transpose1/1
  Mux2/1 -> Transpose2/1
  Transpose2/1 -> PPpose/1
  Bus Selector/2 -> Mux/2, Mux2/2  "<Y>"
  Bus Selector/1 -> Mux/1, Mux2/1  "<X>"

== system ModelForSlidesFeb/Controllers/Subsystem2 ==
  ACCaccel_cmd : Inport
  LCaccel_cmd : Inport  Port=2
  LCdeccel_cmd : Inport  Port=3
  Set Velocity : Inport  Port=4
  ACC : Inport  Port=5
  CurrVelocity : Inport  Port=6
  Relative Distance : Inport  Port=7
  Braking : Inport  Port=8
  CurrAccel : Inport  Port=9
  HoldBrake : Inport  Port=10
  Constant : Constant  Value=0
  MATLAB Function : MATLAB Function  TreatAsAtomicUnit=on
  Subsystem : Subsystem
      settings: PortSchema="{\"entries\":[{\"content\":{\"sides\":[{\"content\":{\"connectorIds\":[\"In1\",\"In2\",\"In3\",\"In4\",\"In5\"]},\"type\":\"ConnectorPlacement.EquallySpacedRectSide\",\"uuid\":\"6c9a9437-5364-4180-a50b-e6d6b79cdde7\"},{\"content\":{\"connectorIds\":[\"Out1\"],\"side\":\"RIGHT\"},\"type\":\"ConnectorPlacement.EquallySpacedRectSide\",\"uuid\":\"0c9d90ab-7b55-4efa-a55f-4d6656a67f49\"},{\"content\":{\"side\":\"TOP\"},\"type\":\"ConnectorPlacement.EquallySpacedRectSide\",\"uuid\":\"ae5230ee-a902-425c-beff-008108cd3a63\"},{\"content\":{\"connectorIds\":[\"In6\"],\"side\":\"BOTTOM\"},\"type\":\"ConnectorPlacement.EquallySpacedRectSide\",\"uuid\":\"84107842-f68a-411d-a329-d9554f488760\"}]},\"type\":\"ConnectorPlacement.EquallySpacedConnector\",\"uuid\":\"1e045dad-e983-4ca4-b515-afd5db4fa0f5\"}],\"packageUris\":[\"http://schema.mathworks.com/mf0/Connector/R2020b\"],\"version\":\"1.0\"}"
  Subsystem1 : Subsystem
  Switch{,1..3} (4 alike) : Switch  Criteria=u2 > Threshold  SaturateOnIntegerOverflow=off  InputSameDT=off
  TorgueCm : Outport
  BrakeCm : Outport  Port=2
  wires:
  Subsystem1/2(brake_cm) -> Switch2/3
  Subsystem1/1(torque_cm) -> Switch3/3
  ACCaccel_cmd/1 -> MATLAB Function/1(u)
  ACC/1 -> Switch1/2, Switch/2
  MATLAB Function/1(accel) -> Switch/1
  LCaccel_cmd/1 -> Switch/3
  Switch/1 -> Subsystem1/1(acc_cmd)
  LCdeccel_cmd/1 -> Switch1/3
  Switch1/1 -> Subsystem1/2(decc_cmd)
  MATLAB Function/2(decel) -> Switch1/1
  Switch2/1 -> BrakeCm/1
  Switch3/1 -> TorgueCm/1
  Constant/1 -> Switch3/1
  Braking/1 -> Switch3/2, Switch2/2, Subsystem/4("Braking ")
  CurrVelocity/1 -> Subsystem/1(CurrVelocity)
  Relative Distance/1 -> Subsystem/2(Relative Distance)
  Subsystem/1(BrakeCm) -> Switch2/1
  CurrAccel/1 -> Subsystem/3(CurrAccel)
  Set Velocity/1 -> Subsystem/5(Set Velocity)
  HoldBrake/1 -> Subsystem/6(HoldBrake)

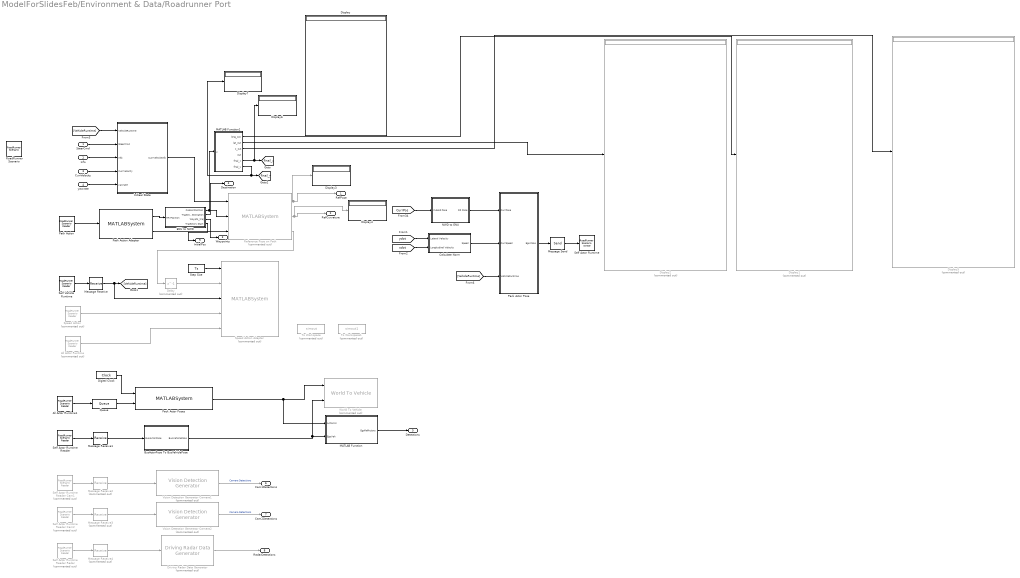
== system ModelForSlidesFeb/Environment & Data/Roadrunner Port ==
  SteerCmd : Inport
  Info : Inport  Port=2
  CurrVelocity : Inport  Port=3
  yawrate : Inport  Port=4
  All Actor Runtime : roadrunnerscenario/RoadRunner Scenario Reader  Commented=on  TopicCategory=Actor  ActorCategory=All Types  ActionType=Path Following  EventType=User-Defined  TopicType=Actor Pose  VehicleType=Vehicle Specifications  UserDefinedAction=Action1  UserDefinedEvent=Event1  Filter=None  SensorTopic=Target Poses  LaneBoundaryOutputTopic=Ego-Lane  SensorID=1  SampleTime=Ts
  All Actor Runtime1 : roadrunnerscenario/RoadRunner Scenario Reader  TopicCategory=Actor  ActorCategory=All Types  ActionType=Path Following  EventType=User-Defined  TopicType=Actor Pose (Driving Scenario compatible)  VehicleType=Vehicle Specifications  UserDefinedAction=Action1  UserDefinedEvent=Event1  Filter=None  SensorTopic=Target Poses  LaneBoundaryOutputTopic=Ego-Lane  SensorID=1  SampleTime=Ts
  BusActorPose To BusVehiclePose : Subsystem
  Calculate Norm : Subsystem
  Delay : Delay  Commented=on  DelayLength=1  InitialCondition=logical(0)
  Digital Clock : DigitalClock  SampleTime=Ts
  Display{,3..4,6..7} (5 alike) : Display
  Display1 : Display  Commented=on
  Display2 : Display  Commented=on
  Display5 : Display  Commented=on
  Driving Radar Data Generator : drivingscenarioandsensors/Driving Radar Data Generator  Commented=on  SensorIndex=1  UpdateRate=100  MountingLocation=[ 3.4, 0, 0.2 ]  MountingAngles=[0 0 0]  HasElevation=off  HasRangeRate=on  HasNoise=on  HasFalseAlarms=on  HasOcclusion=on  MaxNumReportsSource=Property  MaxNumReports=50  TargetReportFormat=Detections  DetectionCoordinates=Body  TrackCoordinates=Body  BusNameSource=Auto  BusName=BusDrivingRadarDataGenerator  AzimuthResolution=4  ElevationResolution=5  RangeResolution=1  RangeRateResolution=0.5  AzimuthBiasFraction=0.1  ElevationBiasFraction=0.1  RangeBiasFraction=0.05  RangeRateBiasFraction=0.05  FieldOfView=[ 180, 5 ]  RangeLimits=[ 0, 150 ]  RangeRateLimits=[ -100, 100 ]  DetectionProbability=1  FalseAlarmRate=1e-06  ReferenceRange=100  ReferenceRCS=0  CenterFrequency=77e9  FilterInitializationFcn=initcvekf  ConfirmationThreshold=[2 3]  DeletionThreshold=[5 5]  InitialSeedSource=Repeatable  InitialSeed=0  UsedSeed=matlabshared.tracking.internal.SimulinkUtilities.seedManager(gcb)  ProfilesSource=MATLAB expression  ProfilesParameters=driving.internal.ActorProfilesRadarParameters  ProfilesExpression=actorProfiles
  ENU to NWD : Subsystem
  Initiaal State : Subsystem
  MATLAB Function : MATLAB Function  TreatAsAtomicUnit=on
  MATLAB Function1 : MATLAB Function  TreatAsAtomicUnit=on
  Message Receive : Receive  InputPortMessageModes=m
  Message Receive1 : Receive  InputPortMessageModes=m  SampleTime=Ts
  Message Receive2 : Receive  Commented=on  InputPortMessageModes=m  SampleTime=Ts
  Message Receive3 : Receive  Commented=on  InputPortMessageModes=m  SampleTime=Ts
  Message Receive4 : Receive  Commented=on  InputPortMessageModes=m  SampleTime=Ts
  Message Send : Send  OutputPortMessageModes=m
  NWD to ENU : Subsystem
  Pack Actor Pose : Subsystem
  Pack Actor Poses : MATLABSystem  InputPortMessageModes=n,m  System=HelperPackDrivingScenarioPoses  EgoActorID=1  ActorProfiles=struct( 'ActorID', 1, 'ClassID', 1, 'Length', 4.7, 'Width', 1.8, 'Height', 1.4, 'OriginOffset', [ 0, 0, 0 ], 'FrontOverhang', 0, 'RearOverhang', 0, 'Wheelbase', 0, 'Color', [ 0, 0, 0 ] )  DefaultActorPoses="Simulink.Bus.createMATLABStruct( \"BusActors\" )"
      mask Type: HelperPackDrivingScenarioPoses
      mask Display:
      | disp(['HelperPack' char(10) 'DrivingScenarioPoses']);
      | port_label('input',1,'time');
      | port_label('input',2,'msgs');
      | port_label('output',1,'TargetPoses');
  Path Action : roadrunnerscenario/RoadRunner Scenario Reader  TopicCategory=Action  ActorCategory=All Types  ActionType=Path Following  EventType=User-Defined  TopicType=Actor Specifications  VehicleType=Vehicle Specifications  UserDefinedAction=Action1  UserDefinedEvent=Event1  Filter=Self  SensorTopic=Target Poses  LaneBoundaryOutputTopic=Ego-Lane  SensorID=1  SampleTime=Ts
  Path Action Adapter : MATLABSystem  InputPortMessageModes=m  System=HelperPathActionAdapter
      mask Type: HelperPathActionAdapter
      mask Display:
      | disp(['HelperPathActionAdapter' char(10) '' char(10) '']);
      | port_label('input',1,'PathAction');
      | port_label('output',1,'Path');
      | port_label('output',2,'NumPoints');
  Queue : Queue  InputPortMessageModes=m  OutputPortMessageModes=m  OverwriteOldest=on  Capacity=maxNumActors+1
  Reference Pose on Path : MATLABSystem  Commented=on  System=HelperReferencePoseOnPath
      mask Type: HelperReferencePoseOnPath
      mask Display:
      | disp(['HelperReferencePoseOnPath' char(10) '' char(10) '' char(10) '' char(10) '']);
      | port_label('input',1,'PrevVehicleInfo');
      | port_label('input',2,'Trajectory');
      | port_label('input',3,'NumTrajPoints');
      | port_label('output',1,'RefPointOnPath');
      | port_label('output',2,'RefCurvature');
      | port_label('output',3,'IsGoalReached');
  RoadRunner Scenario : roadrunnerscenario/RoadRunner Scenario  UserDefinedActions={}  UserDefinedEvents={}
  Self Actor Runtime : roadrunnerscenario/RoadRunner Scenario Writer  TopicCategory=Actor  ActorCategory=All Types  EventType=Action Complete  UserDefinedEvent=Event1  VehicleType=Vehicle Pose  TopicType=Actor Pose
  Self Actor Runtime Reader : roadrunnerscenario/RoadRunner Scenario Reader  TopicCategory=Actor  ActorCategory=All Types  ActionType=Path Following  EventType=User-Defined  TopicType=Actor Pose (Driving Scenario compatible)  VehicleType=Vehicle Specifications  UserDefinedAction=Action1  UserDefinedEvent=Event1  Filter=Self  SensorTopic=Target Poses  LaneBoundaryOutputTopic=Ego-Lane  SensorID=1  SampleTime=Ts
  Self Actor Runtime Reader Cam1 : roadrunnerscenario/RoadRunner Scenario Reader  Commented=on  TopicCategory=Sensor  ActorCategory=All Types  ActionType=Path Following  EventType=User-Defined  TopicType=Actor Pose (Driving Scenario compatible)  VehicleType=Vehicle Specifications  UserDefinedAction=Action1  UserDefinedEvent=Event1  Filter=Self  SensorTopic=Target Poses  LaneBoundaryOutputTopic=Ego-Lane  SensorID=3  SampleTime=Ts
  Self Actor Runtime Reader Cam2 : roadrunnerscenario/RoadRunner Scenario Reader  Commented=on  TopicCategory=Sensor  ActorCategory=All Types  ActionType=Path Following  EventType=User-Defined  TopicType=Actor Pose (Driving Scenario compatible)  VehicleType=Vehicle Specifications  UserDefinedAction=Action1  UserDefinedEvent=Event1  Filter=Self  SensorTopic=Target Poses  LaneBoundaryOutputTopic=Ego-Lane  SensorID=2  SampleTime=Ts
  Self Actor Runtime Reader Radar : roadrunnerscenario/RoadRunner Scenario Reader  Commented=on  TopicCategory=Sensor  ActorCategory=All Types  ActionType=Path Following  EventType=User-Defined  TopicType=Actor Pose (Driving Scenario compatible)  VehicleType=Vehicle Specifications  UserDefinedAction=Action1  UserDefinedEvent=Event1  Filter=Self  SensorTopic=Target Poses  LaneBoundaryOutputTopic=Ego-Lane  SensorID=1  SampleTime=Ts
  Self Vehicle Runtime : roadrunnerscenario/RoadRunner Scenario Reader  TopicCategory=Actor  ActorCategory=Vehicle  ActionType=Path Following  EventType=User-Defined  TopicType=Actor Specifications  VehicleType=Vehicle Pose  UserDefinedAction=Action1  UserDefinedEvent=Event1  Filter=Self  SensorTopic=Target Poses  LaneBoundaryOutputTopic=Ego-Lane  SensorID=1  SampleTime=Ts
  Speed Action : roadrunnerscenario/RoadRunner Scenario Reader  Commented=on  TopicCategory=Action  ActorCategory=All Types  ActionType=Speed Change  EventType=User-Defined  TopicType=Actor Specifications  VehicleType=Vehicle Specifications  UserDefinedAction=Action1  UserDefinedEvent=Event1  Filter=Self  SensorTopic=Target Poses  LaneBoundaryOutputTopic=Ego-Lane  SensorID=1  SampleTime=Ts
  Speed Action Adapter : MATLABSystem  Commented=on  InputPortMessageModes=n,n,n,m,m  System=HelperSpeedActionAdapter
      mask Type: HelperSpeedActionAdapter
      mask Display:
      | disp(['HelperSpeedActionAdapter' char(10) '' char(10) '']);
      | port_label('input',1,'timestep');
      | port_label('input',2,'stopVehicle');
      | port_label('input',3,'vehicleRuntime');
      | port_label('input',4,'msgSpeedAction');
      | port_label('input',5,'msgAllVehicleRuntime');
      | port_label('output',1,'currentSpeed');
  Step Size : Constant  Value=Ts
  To Workspace : ToWorkspace  Commented=on  VariableName=simout  SaveFormat=Timeseries  SampleTime=-1
  To Workspace1 : ToWorkspace  Commented=on  VariableName=simout1  SaveFormat=Timeseries  SampleTime=-1
  Vision Detection Generator Camera1 : drivingscenarioandsensors/Vision Detection Generator  Commented=on  SensorIndex=3  DetectorOutput=Objects only  UpdateInterval=0.01  LaneUpdateInterval=0.1  SensorLocation=[1.9 0]  Height=1.1  Yaw=-45  Pitch=0  Roll=0  BusNameSource=Auto  BusName=BusObjectDetections  BusName2Source=Auto  BusName2=BusLaneDetections  MaxNumDetectionsSource=Property  MaxNumDetections=10  MaxNumLanesSource=Property  MaxNumLanes=30  DetectionCoordinates=Ego Cartesian  SimulateUsing=Interpreted execution  MaxRange=150  BoundingBoxAccuracy=5  ProcessNoiseIntensity=5  MaxSpeed=100  MaxAllowedOcclusion=0.9  MinObjectImageSize=[2 2]  DetectionProbability=1  FalsePositivesPerImage=0  MinLaneImageSize=[20 3]  LaneBoundaryAccuracy=3  HasNoise=off  InitialSeedSource=Repeatable  InitialSeed=0  UsedSeed=0  ActorProfilesSource=MATLAB expression  ActorProfilesParameters=driving.internal.ActorProfilesParameters  ActorProfilesExpression=actorProfiles  Intrinsics=driving.internal.cameraIntrinsics('FocalLength',[200 800],'PrincipalPoint',[320 240],'ImageSize',[640 480],'RadialDistortion',[0 0],'TangentialDistortion',[0 0],'Skew',0)
  Vision Detection Generator Camera2 : drivingscenarioandsensors/Vision Detection Generator  Commented=on  SensorIndex=2  DetectorOutput=Objects only  UpdateInterval=0.01  LaneUpdateInterval=0.1  SensorLocation=[1.9 0]  Height=1.1  Yaw=45  Pitch=0  Roll=0  BusNameSource=Auto  BusName=BusObjectDetections  BusName2Source=Auto  BusName2=BusLaneDetections  MaxNumDetectionsSource=Property  MaxNumDetections=10  MaxNumLanesSource=Property  MaxNumLanes=30  DetectionCoordinates=Ego Cartesian  SimulateUsing=Interpreted execution  MaxRange=150  BoundingBoxAccuracy=5  ProcessNoiseIntensity=5  MaxSpeed=100  MaxAllowedOcclusion=0.9  MinObjectImageSize=[2 2]  DetectionProbability=1  FalsePositivesPerImage=0  MinLaneImageSize=[20 3]  LaneBoundaryAccuracy=3  HasNoise=off  InitialSeedSource=Repeatable  InitialSeed=0  UsedSeed=0  ActorProfilesSource=MATLAB expression  ActorProfilesParameters=driving.internal.ActorProfilesParameters  ActorProfilesExpression=actorProfiles  Intrinsics=driving.internal.cameraIntrinsics('FocalLength',[200 800],'PrincipalPoint',[320 240],'ImageSize',[640 480],'RadialDistortion',[0 0],'TangentialDistortion',[0 0],'Skew',0)
  World To Vehicle : drivingscenarioandsensors/World To Vehicle  Commented=on  BusNameSource=Auto  BusName=BusWorldToVehicleActors  SimulateUsing=Interpreted execution
  RefPose : Outport
  RefCurvature : Outport  Port=2
  Waypoints : Outport  Port=3
  Destination : Outport  Port=4
  Detections : Outport  Port=5
  Cam1Detections : Outport  Port=6
  Cam2Detections : Outport  Port=7
  RadarDetections : Outport  Port=8
  InitialPos : Outport  Port=9
  tag scope: final_x=global, final_y=global
  wires:
  Delay/1 -> Speed Action Adapter/2
  Reference Pose on Path/3 -> Delay/1
  Path Action Adapter/1 -> ENU to NWD/1(RR Position)
  Step Size/1 -> Speed Action Adapter/1
  Self Vehicle Runtime/1 -> Message Receive/1
  Message Receive/1 -> Speed Action Adapter/3, [VehicleRuntime]
  Path Action Adapter/2 -> Reference Pose on Path/3
  Path Action/1 -> Path Action Adapter/1
  Initiaal State/1(CurrVehicleInfo) -> Reference Pose on Path/1
  [VehicleRuntime] -> Initiaal State/1(VehicleRuntime)
  SteerCmd/1 -> Initiaal State/2(SteerCmd)
  Info/1 -> Initiaal State/3(Info)
  CurrVelocity/1 -> Initiaal State/4(CurrVelocity)
  yawrate/1 -> Initiaal State/5(yawrate)
  Reference Pose on Path/1 -> RefPose/1, Display3/1
  Reference Pose on Path/2 -> RefCurvature/1, Display4/1
  Message Send/1 -> Self Actor Runtime/1
  [CurrPos] -> NWD to ENU/1(Cuboid Pose)
  [ydot] -> Calculate Norm/1(Lateral Velocity)
  [xdot] -> Calculate Norm/2(Longitudinal Velocity)
  Calculate Norm/1(Speed) -> Pack Actor Pose/2(CurrSpeed)
  NWD to ENU/1(RR Pose) -> Pack Actor Pose/1(CurrPose)
  [VehicleRuntime] -> Pack Actor Pose/3(VehicleRuntime)
  Pack Actor Pose/1(Ego Pose) -> Message Send/1
  Pack Actor Poses/1 -> MATLAB Function/1(ActorsIn), World To Vehicle/1
  Queue/1 -> Pack Actor Poses/2
  Digital Clock/1 -> Pack Actor Poses/1
  Self Actor Runtime Reader/1 -> Message Receive1/1
  Message Receive1/1 -> BusActorPose To BusVehiclePose/1(BusActorPose)
  All Actor Runtime1/1 -> Queue/1
  Speed Action/1 -> Speed Action Adapter/4
  All Actor Runtime/1 -> Speed Action Adapter/5
  BusActorPose To BusVehiclePose/1(BusVehiclePose) -> MATLAB Function/2(EgoVeh), World To Vehicle/2
  MATLAB Function/1(EgoRefActors) -> Detections/1
  MATLAB Function1/1(long_out) -> Display1/1
  MATLAB Function1/2(lat_out) -> Display2/1
  MATLAB Function1/3(z_out) -> Display5/1
  MATLAB Function1/5(final_x) -> Display6/1, [final_x]
  MATLAB Function1/6(final_y) -> [final_y], Display7/1
  ENU to NWD/1(Cuboid Position) -> MATLAB Function1/1(u), Reference Pose on Path/2
  ENU to NWD/3(Waypts_traj) -> Waypoints/1
  ENU to NWD/2(Trajectory Destination) -> Destination/1
  Message Receive2/1 -> Vision Detection Generator Camera1/1
  Self Actor Runtime Reader Cam1/1 -> Message Receive2/1
  Self Actor Runtime Reader Cam2/1 -> Message Receive3/1
  Message Receive3/1 -> Vision Detection Generator Camera2/1
  Self Actor Runtime Reader Radar/1 -> Message Receive4/1
  Message Receive4/1 -> Driving Radar Data Generator/1
  Driving Radar Data Generator/1 -> RadarDetections/1
  Vision Detection Generator Camera2/1 -> Cam2Detections/1  "Camera Detections"
  Vision Detection Generator Camera1/1 -> Cam1Detections/1  "Camera Detections"
  ENU to NWD/4(Trajectory Start) -> InitialPos/1

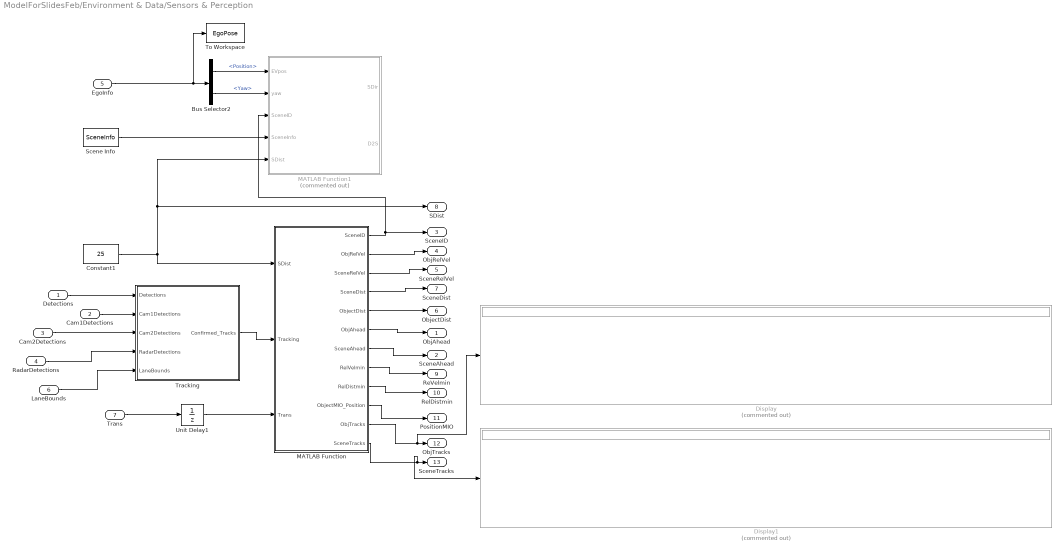
== system ModelForSlidesFeb/Environment & Data/Sensors & Perception ==
  Detections : Inport
  Cam1Detections : Inport  Port=2
  Cam2Detections : Inport  Port=3
  RadarDetections : Inport  Port=4
  EgoInfo : Inport  Port=5
  LaneBounds : Inport  Port=6
  Trans : Inport  Port=7
  Bus Selector2 : BusSelector  OutputSignals=Position,Yaw
  Constant1 : Constant  Value=25
  Display : Display  Commented=on
  Display1 : Display  Commented=on
  MATLAB Function : MATLAB Function  TreatAsAtomicUnit=on
  MATLAB Function1 : MATLAB Function  Commented=on  TreatAsAtomicUnit=on
  Scene Info : Constant  Value=SceneInfo  VectorParams1D=off
  To Workspace : ToWorkspace  VariableName=EgoPose  SaveFormat=Timeseries  SampleTime=-1
  Tracking : Subsystem
  Unit Delay1 : UnitDelay  SampleTime=0.05  HasFrameUpgradeWarning=on
  ObjAhead : Outport
  SceneAhead : Outport  Port=2
  SceneID : Outport  Port=3
  ObjRelVel : Outport  Port=4
  SceneRelVel : Outport  Port=5
  ObjectDist : Outport  Port=6
  SceneDist : Outport  Port=7
  SDist : Outport  Port=8
  ReVelmin : Outport  Port=9
  RelDistmin : Outport  Port=10
  PositionMIO : Outport  Port=11
  ObjTracks : Outport  Port=12
  SceneTracks : Outport  Port=13
  wires:
  MATLAB Function/6(ObjAhead) -> ObjAhead/1
  MATLAB Function/5(ObjectDist) -> ObjectDist/1
  MATLAB Function/7(SceneAhead) -> SceneAhead/1
  MATLAB Function/2(ObjRelVel) -> ObjRelVel/1
  EgoInfo/1 -> To Workspace/1, Bus Selector2/1
  Bus Selector2/1 -> MATLAB Function1/1(EVpos)  "<Position>"
  Detections/1 -> Tracking/1(Detections)
  Scene Info/1 -> MATLAB Function1/4(SceneInfo)
  Bus Selector2/2 -> MATLAB Function1/2(yaw)  "<Yaw>"
  Tracking/1(Confirmed_Tracks) -> MATLAB Function/2(Tracking)
  Constant1/1 -> MATLAB Function1/5(SDist), SDist/1, MATLAB Function/1(SDist)
  MATLAB Function/1(SceneID) -> MATLAB Function1/3(SceneID), SceneID/1
  MATLAB Function/4(SceneDist) -> SceneDist/1
  MATLAB Function/3(SceneRelVel) -> SceneRelVel/1
  MATLAB Function/8(RelVelmin) -> ReVelmin/1
  MATLAB Function/9(RelDistmin) -> RelDistmin/1
  Trans/1 -> Unit Delay1/1
  Unit Delay1/1 -> MATLAB Function/3(Trans)
  LaneBounds/1 -> Tracking/5(LaneBounds)
  MATLAB Function/10(ObjectMIO_Position) -> PositionMIO/1
  MATLAB Function/11(ObjTracks) -> Display/1, ObjTracks/1
  MATLAB Function/12(SceneTracks) -> Display1/1, SceneTracks/1
  Cam1Detections/1 -> Tracking/2(Cam1Detections)
  Cam2Detections/1 -> Tracking/3(Cam2Detections)
  RadarDetections/1 -> Tracking/4(RadarDetections)

== system ModelForSlidesFeb/Environment & Data/Subsystem1 ==
  VehFdbk : Inport
  Bus Selector : BusSelector  OutputSignals=InertFrm.Cg.Disp.X,InertFrm.Cg.Disp.Y,InertFrm.Cg.Ang.psi
  Gain1 : Gain  Gain=180/pi
  Mux : Mux  Inputs=3
  Transpose : Math  Operator=transpose  SignedPower=on
  pose : Outport
  wires:
  Mux/1 -> Transpose/1
  VehFdbk/1 -> Bus Selector/1
  Gain1/1 -> Mux/3
  Transpose/1 -> pose/1
  Bus Selector/3 -> Gain1/1  "<psi>"
  Bus Selector/2 -> Mux/2  "<Y>"
  Bus Selector/1 -> Mux/1  "<X>"
